simulink library "tetherInternalForcesNGreater2_ul"  (R2018b)
settings: Solver=VariableStepAuto  StartTime=0.0  StopTime=10.0  RelTol=1e-3
values from neighbouring files (symbols this model uses):
  E = 3.8e9    (= 3800000000)    [tetherInternalForces_ts.m]
  mass = 100    [tetherInternalForces_ts.m]
  N = 2    [tetherInternalForces_ts.m]
  zeta = 0.05    [tetherInternalForces_ts.m]
settings Model: Creator=asiddiq2  LastModifiedBy=asiddiq2

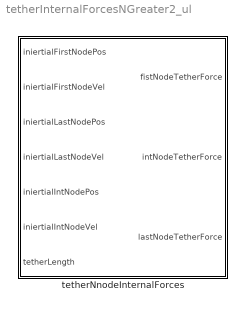
== system tetherInternalForcesNGreater2_ul ==
  tetherNnodeInternalForces : Subsystem  mask{massBdy=mass, numNode=N, diaTether=0, youngsTether=E, zetaTether=zeta}
      mask prompts: massBdy "Vehicle Mass (kg)"; numNode "Number of nodes"; diaTether "Tether diameter"; youngsTether "Youngs Modulus"; zetaTether "Damping ratio"
      mask DialogControl Container3 Prompt: Vehicle

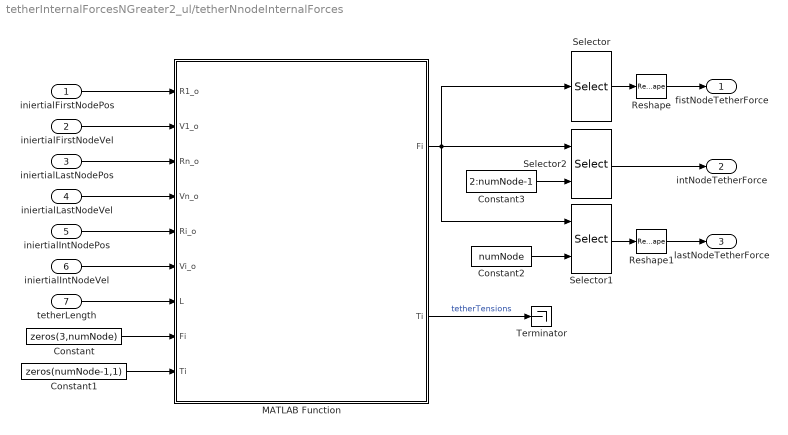
== system tetherInternalForcesNGreater2_ul/tetherNnodeInternalForces ==
  iniertialFirstNodePos : Inport
  iniertialFirstNodeVel : Inport  Port=2
  iniertialLastNodePos : Inport  Port=3
  iniertialLastNodeVel : Inport  Port=4
  iniertialIntNodePos : Inport  Port=5
  iniertialIntNodeVel : Inport  Port=6
  tetherLength : Inport  Port=7
  Constant : Constant  Value=zeros(3,numNode)  VectorParams1D=off
  Constant1 : Constant  Value=zeros(numNode-1,1)  VectorParams1D=off
  Constant2 : Constant  Value=numNode  VectorParams1D=off
  Constant3 : Constant  Value=2:numNode-1  VectorParams1D=off
  MATLAB Function : MATLAB Function  TreatAsAtomicUnit=on
  Reshape : Reshape  OutputDimensionality=Column vector (2-D)
  Reshape1 : Reshape  OutputDimensionality=Column vector (2-D)
  Selector : Selector  NumberOfDimensions=2  InputPortWidth=3  IndexOptions=Select all,Index vector (dialog)  Indices=[1 3],1  OutputSizes=1,1
  Selector1 : Selector  NumberOfDimensions=2  InputPortWidth=3  IndexOptions=Select all,Index vector (port)  Indices=[1 3],N  OutputSizes=1,1
  Selector2 : Selector  NumberOfDimensions=2  InputPortWidth=3  IndexOptions=Select all,Index vector (port)  Indices=[1 3],[2:N-1]  OutputSizes=1,1
  Terminator : Terminator
  fistNodeTetherForce : Outport
  intNodeTetherForce : Outport  Port=2
  lastNodeTetherForce : Outport  Port=3
  wires:
  MATLAB Function/2(Ti) -> Terminator/1  "tetherTensions"
  iniertialLastNodePos/1 -> MATLAB Function/3(Rn_o)
  iniertialLastNodeVel/1 -> MATLAB Function/4(Vn_o)
  iniertialIntNodePos/1 -> MATLAB Function/5(Ri_o)
  iniertialIntNodeVel/1 -> MATLAB Function/6(Vi_o)
  iniertialFirstNodePos/1 -> MATLAB Function/1(R1_o)
  iniertialFirstNodeVel/1 -> MATLAB Function/2(V1_o)
  tetherLength/1 -> MATLAB Function/7(L)
  Constant/1 -> MATLAB Function/8("Fi ")
  Constant1/1 -> MATLAB Function/9("Ti ")
  Selector1/1 -> Reshape1/1
  Selector2/1 -> intNodeTetherForce/1
  MATLAB Function/1(Fi) -> Selector2/1, Selector1/1, Selector/1
  Constant2/1 -> Selector1/2
  Constant3/1 -> Selector2/2
  Selector/1 -> Reshape/1
  Reshape/1 -> fistNodeTetherForce/1
  Reshape1/1 -> lastNodeTetherForce/1

== matlab function tetherInternalForcesNGreater2_ul/tetherNnodeInternalForces/MATLAB Function ==
  data: R1_o input; V1_o input; Rn_o input; Vn_o input; Fi output; Ri_o input; Vi_o input; L input; Fi input; Ti input; numNode parameter; massBdy parameter; zetaTether parameter; youngsTether parameter; Ti output; diaTether parameter
 function [Fi,Ti]  = fcn(R1_o,V1_o,Rn_o,Vn_o,Ri_o,Vi_o,L,Fi,Ti,...
     numNode, massBdy, zetaTether, youngsTether, diaTether)

Ri_o = [R1_o Ri_o Rn_o];
Vi_o = [V1_o Vi_o Vn_o];
 
% cross sectional area
CS = (pi/4)*diaTether^2;

% total spring stiffness
k_tot = youngsTether*CS/L;

% total damping coefficient
c_tot = zetaTether*2*sqrt(k_tot*massBdy);

% inidividual spring stiffness and damping
k = k_tot*(numNode-1);
c = c_tot*(numNode-1);
Li = L/(numNode-1);

% determine distance between nodes and the derivatives of each element
di = zeros(numNode-1,1);
direction = zeros(3,numNode-1);
di_dot = zeros(numNode-1,1);
Tk = zeros(numNode-1,1);
Td = zeros(numNode-1,1);
F_t_i = zeros(3,numNode);


for ii = 1:numNode-1
        di(ii) = norm(Ri_o(:,ii+1) - Ri_o(:,ii));
        direction(:,ii) = (Ri_o(:,ii+1) - Ri_o(:,ii))/di(ii);
        di_dot(ii) = dot(Ri_o(:,ii+1) - Ri_o(:,ii),Vi_o(:,ii+1) - Vi_o(:,ii))/di(ii);
    
end

% spring and damper forces
for ii = 1:numNode-1
    if di(ii) > Li
        Tk(ii) = k*(di(ii) - Li);
        Td(ii) = c*di_dot(ii);
        F_t_i(:,ii) = (Tk(ii) + Td(ii))*direction(:,ii);
        Ti(ii) = norm(F_t_i(:,ii));
    else
        Tk(ii) = 0;
        Td(ii) = 0;
        F_t_i(:,ii) = (Tk(ii) + Td(ii))*direction(:,ii);
        Ti(ii) = norm(F_t_i(:,ii));

    end
end

for ii = 1:numNode
    if ii == 1
        Fi(:,ii) = F_t_i(:,ii);
    elseif ii > 1 && ii < numNode
        Fi(:,ii) = F_t_i(:,ii) - F_t_i(:,ii-1);
    elseif ii == numNode
        Fi(:,ii) = -F_t_i(:,ii-1);
    end
end


% Mitchells version here (Should be equivalen to almost all of the above)
%  di = sqrt(sum(diff(Ri_o,1,2).^2,1))';
%  direction = diff(Ri_o,1,2)./repmat(di',[N-1 1]);
%  di_dot = sum(direction.*diff(Vi_o,1,2),1)';
%  Tk(di>Li) = k*(di(di>Li) - Li)
%  Td(di>Li) = c*di_dot(di>Li)
%  F_t_i(1:end-1) = repmat((Tk' + Td'),[N-1 1]).*direction


end
